simulink model "SCARA_Ass5_Arm_Control"  (Simulink 7.4)
settings: Solver=FixedStepDiscrete  StartTime=0.0  StopTime=inf  FixedStep=0.00001  RelTol=1e-3
libraries: simulink x1, RT x1, vrlib x1
settings Model: Creator=Mengchen  LastModifiedBy=t6z8
settings OptimizationCC: ExpressionDepthLimit=128  InitFltsAndDblsToZero=on
settings DebuggingCC: AlgebraicLoopMsg=error  SaveWithParameterizedLinksMsg=none  StateNameClashWarn=none  StrictBusMsg=ErrorLevel1
settings HardwareCC: TargetEndianess=LittleEndian  TargetHWDeviceType=MATLAB Host
settings RTWCC: ProcessScript=grt_make_rtw_hook  CustomHeaderCode="#include \"haptics.h\""  CustomInclude="\"C:\\Program Files\\novint\\HDAL_SDK_1.1.0_Beta\\include\""  TargetLang=C++
settings CodeAppCC: CustomSymbolStrType=$N$R$M_T

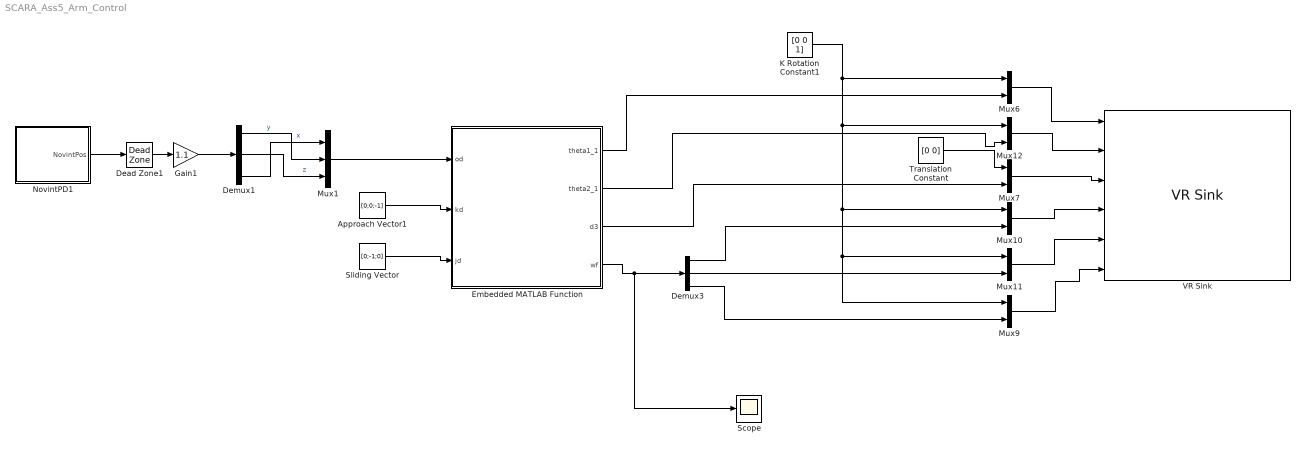
== system SCARA_Ass5_Arm_Control ==
  Approach Vector1 : Constant  Value=[0;0;-1]
  Dead Zone1 : DeadZone  SaturateOnIntegerOverflow=on
  Demux1 : Demux  Outputs=3
  Demux3 : Demux  Outputs=3
  Embedded MATLAB Function : Stateflow chart
  Gain1 : Gain  Gain=1.1  ParameterDataType=fixdt(1, 16)  ParameterScaling=2^0  OutDataType=fixdt(1, 16)  OutScaling=2^0
  K Rotation Constant1 : Constant  Value=[0 0 1]
  Mux1 : Mux  Inputs=3
  Mux{6..7,9..12} (6 alike) : Mux  Inputs=2
  NovintPD1 : Subsystem
  Scope : Scope
      settings: SaveName=ScopeData3
  Sliding Vector : Constant  Value=[0;-1;0]
  Translation Constant : Constant  Value=[0 0]
  VR Sink : vrlib/VR Sink  InstantiateOnLoad=on  SampleTime=-1  ViewEnable=on  RemoteChange=off  RemoteView=on  FieldsWritten=Link_0_Rotation.rotation.4.1.double#Link_1_Rotation.rotation.4.1.double#Link_2_Translation.translation.3.1.double#Link_3_Rotation.rotation.4.1.double#Link_4_Rotation.rotation.4.1.double#Link_5_Rotation.rotation.4.1.double  WorldFileName=SCARAWORLD.WRL  AutoView=off  VideoDimensions=[]
  wires:
  K Rotation Constant1/1 -> Mux6/1, Mux10/1, Mux11/1, Mux9/1, Mux12/1
  Mux6/1 -> VR Sink/1
  Mux7/1 -> VR Sink/3
  Translation Constant/1 -> Mux7/1
  Mux10/1 -> VR Sink/4
  Mux11/1 -> VR Sink/5
  Mux9/1 -> VR Sink/6
  Mux12/1 -> VR Sink/2
  Embedded MATLAB Function/1(theta1_1) -> Mux6/2
  Embedded MATLAB Function/2(theta2_1) -> Mux12/2
  Embedded MATLAB Function/3(d3) -> Mux7/2
  Demux3/1 -> Mux10/2
  Demux3/2 -> Mux11/2
  Demux3/3 -> Mux9/2
  Embedded MATLAB Function/4(wf) -> Demux3/1, Scope/1
  Approach Vector1/1 -> Embedded MATLAB Function/2(kd)
  Sliding Vector/1 -> Embedded MATLAB Function/3(jd)
  Dead Zone1/1 -> Gain1/1
  NovintPD1/1(NovintPos) -> Dead Zone1/1
  Demux1/1 -> Mux1/2  "y"
  Demux1/2 -> Mux1/3  "z"
  Demux1/3 -> Mux1/1  "x"
  Gain1/1 -> Demux1/1
  Mux1/1 -> Embedded MATLAB Function/1(od)

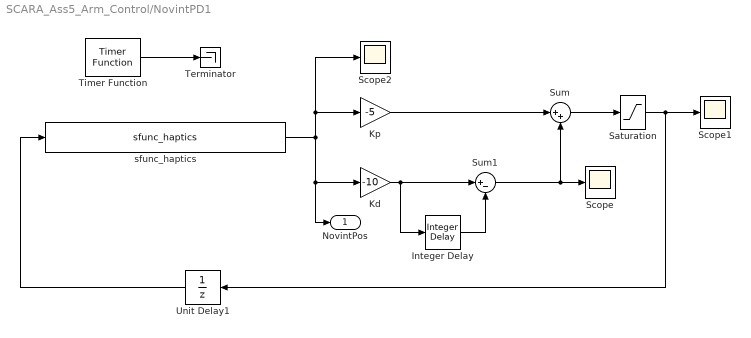
== system SCARA_Ass5_Arm_Control/NovintPD1 ==
  Integer Delay : simulink/Discrete/Integer Delay  vinit=0.0  samptime=-1  NumDelays=2
  Kd : Gain  Gain=-10
  Kp : Gain  Gain=-5
  Saturation : Saturate  UpperLimit=200  LowerLimit=-200
  Scope : Scope
      settings: YMin=-0.9  YMax=0.6
  Scope1 : Scope
  Scope2 : Scope
      settings: YMin=-1.2  YMax=1  SaveName=ScopeData2
  Sum : Sum  Inputs=|++
  Sum1 : Sum  Inputs=|+-
  Terminator : Terminator
  Timer Function : RT/Timer Function  step1=0.9  priority1=HIGH  ThPriority1=TIME CRITICAL
  Unit Delay1 : UnitDelay  SampleTime=-1
  sfunc_haptics : S-Function  FunctionName=sfunc_haptics  EnableBusSupport=off  mask(Legacy Function){SFunctionSpec=void falconPlant(double u1[3], double y1[3]), ShowSpec=on}
      mask prompts: ShowSpec "Display function specification"
      mask help:
      | This block allows you to call the legacy functions specified by the following Legacy Code Tool definition:
      | def.SFunctionName = 'sfunc_haptics';
      | def.OutputFcnSpec = 'void falconPlant(double u1[3], double y1[3])';
      | def.StartFcnSpec = 'createHaptics()';
      | def.TerminateFcnSpec = 'deleteHaptics()';
      | def.HeaderFiles = {'haptics.h'};
      | def.SourceFiles = {'haptics.cpp'};
      | def.HostLibFiles = {'hdl.lib'};
      | def.TargetLibFiles = {'hdl.lib'};
      | def.IncPaths = {'C:\Program Files (x86)\novint\HDAL_SDK_2.1.3\include'};
      | def.LibPaths = {'C:\Program Files (x86)\novint\HDAL_SDK_2.1.3\lib'};
      | def.Options.useTlcWithAccel = false;
      | def.Options.language = 'C++';
      mask Help: <p>This block was generated automatically by the Legacy Code Tool. For detailed help on this tool, call<a href="matlab:legacy_code('help')"> legacy_code('help')</a>.</p>
      mask CallbackString:
      | |if strcmp(get_param(gcbh, 'ShowSpec'), 'on')
      |   set_param(gcbh, 'MaskDisplay', sprintf('fprintf(''%s'');', get_param(gcbh, 'SFunctionSpec')));
      | else
      |   set_param(gcbh, 'MaskDisplay', sprintf('fprintf(''%s'');', get_param(gcbh, 'FunctionName')));
      | end
      mask Display: fprintf('void falconPlant(double u1[3], double y1[3])');
  NovintPos : Outport
  wires:
  Saturation/1 -> Scope1/1, Unit Delay1/1
  Sum/1 -> Saturation/1
  Kp/1 -> Sum/1
  Sum1/1 -> Sum/2, Scope/1
  Integer Delay/1 -> Sum1/2
  Kd/1 -> Sum1/1, Integer Delay/1
  Unit Delay1/1 -> sfunc_haptics/1
  sfunc_haptics/1 -> Kp/1, Scope2/1, NovintPos/1, Kd/1
  Timer Function/1 -> Terminator/1

== matlab function Embedded MATLAB Function ==
  data: od input double; theta1_1 output double; theta2_1 output double; d3 output double; kd input double; jd input double; wf output double
function [theta1_1, theta2_1, d3, wf] = hw5_inverse_function(od, kd, jd)

l1 = 1;
l2 = 1;
l3 = 0.5;
l6 = 0.2;

i = [1; 0; 0];
j = [0; 1; 0];
k = [0; 0; 1];

kx = [0 0 0;
      0 0 -1;
      0 1 0];

o0 = [0; 0; 0];
C0 = eye(3);

coord0 = [C0 o0;
          zeros(1,3) 1];

% Ask for o6, approach vector and sliding vector
%od = input('Enter od ([od_i; od_j; od_k]): ');
%kd = input('Enter approach vector (kd) ([kd_i; kd_j; kd_k]): ');
%jd = input('Enter sliding vector (jd) ([jd_i; jd_j; jd_k]): ');
id = -cross(kd, jd);

Cd = [id jd kd];

% Calculate wrist center

o3 = od - Cd*l6*k;

o2 = o3;

o2(3) = l3+l6;

d3 = o2(3) - o3(3) - l3;

% Solve inverse arm kinematics
% see Slide 1 of Inverse Kinematics slides
u = o2 - o0;
l = sqrt(u(1)*u(1) + u(2)*u(2));

theta2_1 = pi - acos((-l^2 + l1^2 + l2^2)/(2*l1*l2));

alpha = atan(-u(1)/u(2));

% the atan always returns a value between -pi/2 and pi/2,
% so you have to check if the point you want to reach is in the left half
if u(2) < 0
    alpha = alpha + pi;
end

beta = acos((-l2^2 + l1^2 + l^2)/(2*l1*l));

theta1_1 = alpha - beta;

% other solution

%theta1_2 = alpha + beta;
%theta2_2 = -theta2_1;

% there are infinte solutions for theta1 if the gripper is supposed
% to be at the origin ([0; 0; 0])
if isnan(u(1)/u(2))
    %disp('Infinite solutions for theta1, just displaying one with theta1 = 0');
    theta1_1 = 0;
    theta2_1 = pi;
    
    %theta1_2 = 0;
    %theta2_2 = pi;
end

%a1 = [ (theta1_1* (pi / 180)), (theta2_1* (pi / 180)), d3];
%a1 = [a1;a1];
%a2 = [ theta1_2, theta2_2, d3];
%a2 = [a2;a2];

% Get wrist base frame by direct kinematics
coord3_1 = solve_arm_forward(coord0, theta1_1, theta2_1, d3);
%coord3_2 = solve_arm_forward(coord0, theta1_2, theta2_2, d3);

w1 = solve_wrist_inverse(coord3_1,  od, kd, jd);
wf=w1(2,:);
%w2 = solve_wrist_inverse(coord3_2,  od, kd, jd);

%result = [ a1 w1; a2 w2]
